simulink model "LQG_test"  (R2015a)
settings: Solver=ode5  StartTime=0.0  StopTime=14  FixedStep=1e-4  RelTol=1e-3
values from neighbouring files (symbols this model uses):
  Ap = Ap(1:4,1:4)    [main_matlab.m]
  Bp = Bp(1:4,:)    [main_matlab.m]
  Cp = Cp(:,1:4)    [main_matlab.m]
  Hp = Hp(1:4,:)    [main_matlab.m]
libraries: simulink x1, cstblocks x1
settings Model: Creator=p4wp4w  LastModifiedBy=p4wp4w

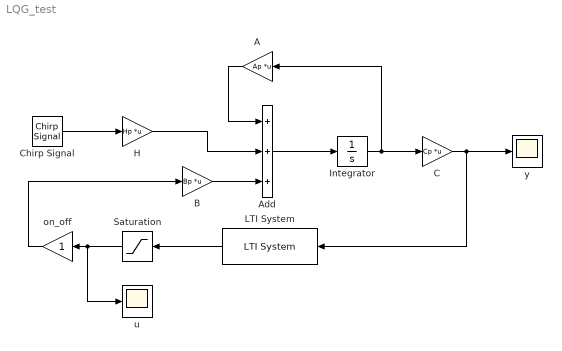
== system LQG_test ==
  A : Gain  Gain=Ap  Multiplication=Matrix(K*u)
  Add : Sum  Inputs=+++
  B : Gain  Gain=Bp  Multiplication=Matrix(K*u)
  C : Gain  Gain=Cp  Multiplication=Matrix(K*u)
  Chirp Signal : simulink/Sources/Chirp Signal  f1=0.1  T=14  f2=140
  H : Gain  Gain=Hp  Multiplication=Matrix(K*u)
  Integrator : Integrator
  LTI System : cstblocks/LTI System  sys=rlqg  IC=[]
  Saturation : Saturate  UpperLimit=1.5  LowerLimit=-1.5
  on_off : Gain
  u : Scope
  y : Scope
  wires:
  Add/1 -> Integrator/1
  A/1 -> Add/1
  B/1 -> Add/3
  Integrator/1 -> C/1, A/1
  C/1 -> y/1, LTI System/1
  LTI System/1 -> Saturation/1
  H/1 -> Add/2
  Chirp Signal/1 -> H/1
  on_off/1 -> B/1
  Saturation/1 -> u/1, on_off/1
